simulink model "P1"  (R2020b)
settings: Solver=VariableStepAuto  StartTime=0.0  StopTime=10.0  RelTol=1e-3
settings Model: Creator=ASUS  LastModifiedBy=ASUS

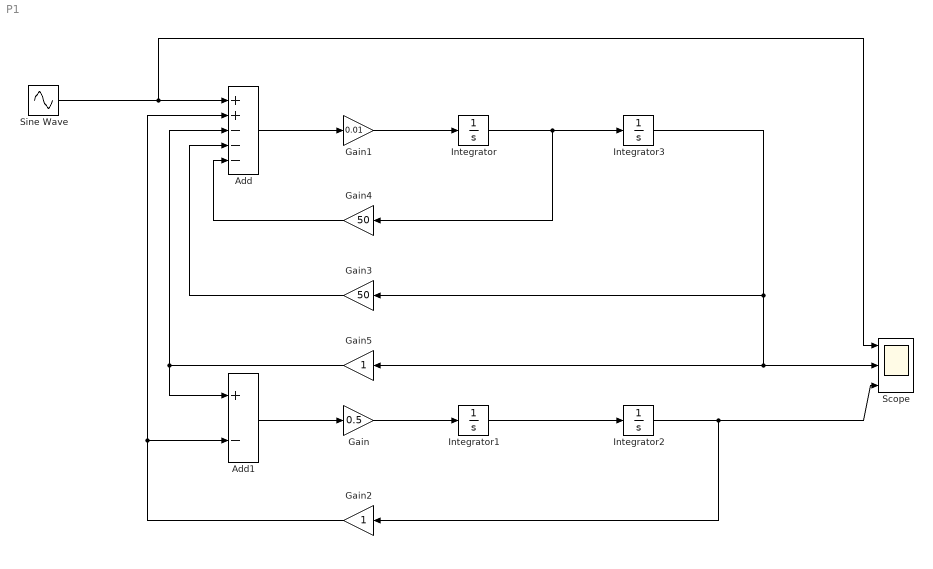
== system P1 ==
  Add : Sum  Inputs=++---
  Add1 : Sum  Inputs=+-
  Gain : Gain  Gain=0.5
  Gain1 : Gain  Gain=0.01
  Gain2 : Gain
  Gain3 : Gain  Gain=50
  Gain4 : Gain  Gain=50
  Gain5 : Gain
  Integrator{,1..3} (4 alike) : Integrator
  Scope : Scope  NumInputPorts=3
  Sine Wave : Sin  Frequency=10  SampleTime=2*10^-4
  wires:
  Integrator/1 -> Gain4/1, Integrator3/1
  Sine Wave/1 -> Add/1, Scope/1
  Integrator1/1 -> Integrator2/1
  Gain/1 -> Integrator1/1
  Add1/1 -> Gain/1
  Add/1 -> Gain1/1
  Gain1/1 -> Integrator/1
  Gain4/1 -> Add/5
  Gain3/1 -> Add/4
  Gain5/1 -> Add/3, Add1/1
  Gain2/1 -> Add/2, Add1/2
  Integrator3/1 -> Gain5/1, Scope/2, Gain3/1
  Integrator2/1 -> Scope/3, Gain2/1
